simulink model "CAR_Simulink"  (R2016a)
settings: Solver=FixedStepDiscrete  StartTime=0.0  StopTime=inf  FixedStep=0.1  RelTol=1e-3
libraries: arduinolib x7
settings Model: SimulationMode=external  ExtModeTrigDuration=2  Creator=pc  LastModifiedBy=pc
settings SolverCC: AutoInsertRateTranBlk=on
settings DataIOCC: LimitDataPoints=on
settings OptimizationCC: OptimizeModelRefInitCode=on  LifeSpan=1  MaxStackSize=64
settings DebuggingCC: AllowSymbolicDim=off
settings HardwareCC: ProdBitPerInt=16  ProdBitPerPointer=16  ProdLargestAtomicFloat=None  ProdWordSize=8  ProdHWDeviceType=Atmel->AVR
settings RTWCC: SystemTargetFile=ert.tlc  HardwareBoard=Arduino Uno  TemplateMakefile=ert_default_tmf  GenerateReport=on  Toolchain=Arduino AVR v1.6.1  BuildConfiguration=Faster Runs  IncludeHyperlinkInReport=on  LaunchReport=on  GenerateTraceInfo=on  GenerateTraceReport=on  GenerateTraceReportSl=on  GenerateTraceReportSf=on  GenerateTraceReportEml=on
settings CodeAppCC: ForceParamTrailComments=on  IgnoreCustomStorageClasses=off  OperatorAnnotations=on  SimulinkDataObjDesc=on  SFDataObjDesc=on  MATLABFcnDesc=on  InsertBlockDesc=on  MATLABSourceComments=on
settings ERTTargetCC: SupportContinuousTime=on  SupportVariableSizeSignals=on
settings ConfigComp: CovModelRefEnable=Off  CovSFcnEnable=off

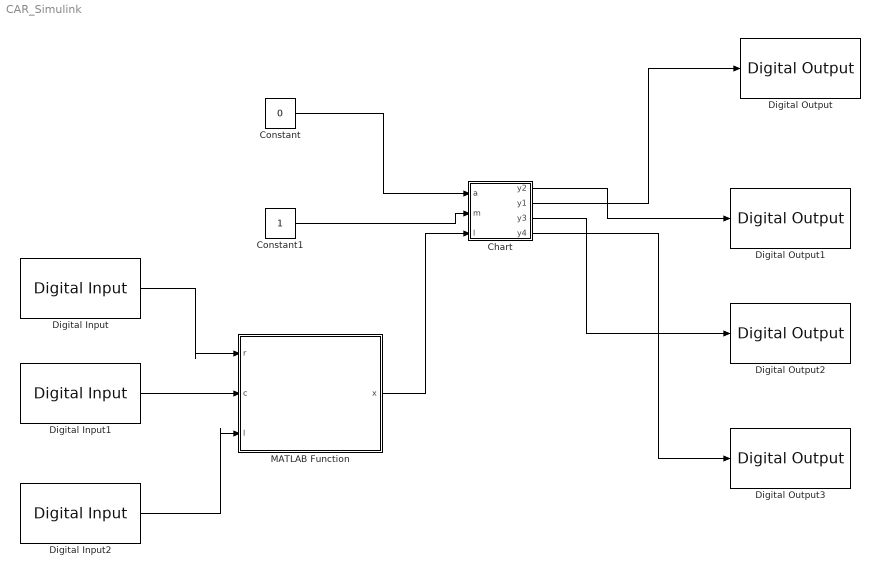
== system CAR_Simulink ==
  Chart : Stateflow chart  TreatAsAtomicUnit=on
  Constant : Constant  Value=0
  Constant1 : Constant
  Digital Input : arduinolib/Digital Input  pinNumber=3  sampleTime=1  blockPlatform=arduino
  Digital Input1 : arduinolib/Digital Input  pinNumber=4  sampleTime=1  blockPlatform=arduino
  Digital Input2 : arduinolib/Digital Input  pinNumber=5  sampleTime=1  blockPlatform=arduino
  Digital Output : arduinolib/Digital Output  pinNumber=8  blockPlatform=arduino
  Digital Output1 : arduinolib/Digital Output  pinNumber=9  blockPlatform=arduino
  Digital Output2 : arduinolib/Digital Output  pinNumber=10  blockPlatform=arduino
  Digital Output3 : arduinolib/Digital Output  pinNumber=11  blockPlatform=arduino
  MATLAB Function : MATLAB Function  TreatAsAtomicUnit=on
  wires:
  Chart/2(y1) -> Digital Output/1
  Chart/1(y2) -> Digital Output1/1
  Chart/3(y3) -> Digital Output2/1
  Constant/1 -> Chart/1(a)
  Chart/4(y4) -> Digital Output3/1
  Digital Input/1 -> MATLAB Function/1(r)
  Constant1/1 -> Chart/2(m)
  Digital Input1/1 -> MATLAB Function/2(c)
  Digital Input2/1 -> MATLAB Function/3(l)
  MATLAB Function/1(x) -> Chart/3(l)

== matlab function CAR_Simulink/MATLAB Function ==
  data: r input; x output; c input; l input
function x  = fcn(r,c,l)
%#codegen

if (l==0 && c==1 && r ==0)   % fwd
    x=1;

elseif (l==0 && c==0 && r ==0)  % stop
    x=2;
    
elseif (l==0 && c==0 && r ==1)  % right 
   x=3;
   
elseif (l==1 && c==0 && r ==0)  %left
    x=4;
else
    x=1;
    
end

    


end

== stateflow chart CAR_Simulink/Chart ==
  state MODE
    entry: y1=0
    y2=0
    y3=0
    y4=0
  state stop
    entry: y1=0
    y2=0
    y3=0
    y4=0
  state m1
    entry: y1= 5
    y3=5
    y2=0
    y4=0
  state m4
    entry: y1=5
    y2=0
    y3=0
    y4=0
  state m3
    entry: y3=5
    y1=0
    y2=0
    y4=0
  state m2
    entry: y2=5
    y4=5
    y1=0
    y3=0
  state LineFollower
    entry: y1=0
    y2=0
    y3=0
    y4=0
  state LEFT
    entry: y1=5
    y2=0
    y3=0
    y4=0
  state RIGHT1
    entry: y3=5
    y1=0
    y2=0
    y4=0
  state STOP
    entry: y2=0
    y4=0
    y1=0
    y3=0
  state FWD
    entry: y1= 5
    y3=5
    y2=0
    y4=0
  (default) -> MODE
  MODE -> stop [order 2] : [m==1]
  MODE -> LineFollower [order 1] : [m==2]
  m4 -> m1 [order 1] : [a==1  && m==1]
  m2 -> m3 [order 1] : [a==3 && m==1]
  stop -> MODE [order 2] : [m==2]
  STOP -> MODE [order 4] : [m==1]
  m3 -> m4 [order 1] : [a==4 && m==1]
  stop -> m1 [order 1] : [a==1 && m==1]
  m3 -> m2 [order 2] : [a==2 && m==1]
  m1 -> m2 [order 1] : [a==2 && m==1]
  LineFollower -> LEFT [order 4] : [l==4]
  LineFollower -> RIGHT1 [order 3] : [l==3]
  LineFollower -> STOP [order 2] : [l==2]
  m3 -> stop [order 4] : [a==0 && m==1]
  m3 -> m1 [order 3] : [a==1 && m==1]
  m1 -> m3 [order 2] : [a==3 && m==1]
  m4 -> m3 [order 2] : [a==3 && m==1]
  m4 -> stop [order 4] : [a==0 && m==1]
  m1 -> m4 [order 3] : [a==4 && m==1]
  m2 -> m4 [order 3] : [a==4 && m==1]
  m4 -> m2 [order 3] : [a==2 && m==1]
  LineFollower -> FWD [order 1] : [l==1]
  m2 -> stop [order 4] : [a==0 && m==1]
  m1 -> stop [order 4] : [a==0 && m==1]
  m2 -> m1 [order 2] : [a==1 && m==1]
  LEFT -> STOP [order 2] : [l==2]
  RIGHT1 -> STOP [order 2] : [l==2]
  FWD -> STOP [order 1] : [l==2]
  RIGHT1 -> FWD [order 1] : [l==1]
  FWD -> RIGHT1 [order 2] : [l==3]
  STOP -> RIGHT1 [order 2] : [l==3]
  LEFT -> RIGHT1 [order 3] : [l==3]
  RIGHT1 -> LEFT [order 3] : [l==4]
  STOP -> FWD [order 1] : [l==1]
  FWD -> LEFT [order 3] : [l==4]
  LEFT -> FWD [order 1] : [l==1]
  STOP -> LEFT [order 3] : [l==4]
  data: y2 output; y1 output; y3 output; y4 output; a input; m input; l input
